simulink model "Single_Phase_FLL"  (R2021b)
settings: Solver=VariableStepAuto  StartTime=0.0  StopTime=2  RelTol=1e-3
libraries: dspswit3 x2, spsThreePhaseProgrammableVoltageSourceLib x1, spsThreePhaseVIMeasurementLib x1, spspowerguiLib x1
settings Model: Creator=Swaran Pratap Singh  LastModifiedBy=Swaran Pratap Singh
settings DataIOCC: InspectSignalLogs=on  ReturnWorkspaceOutputs=off

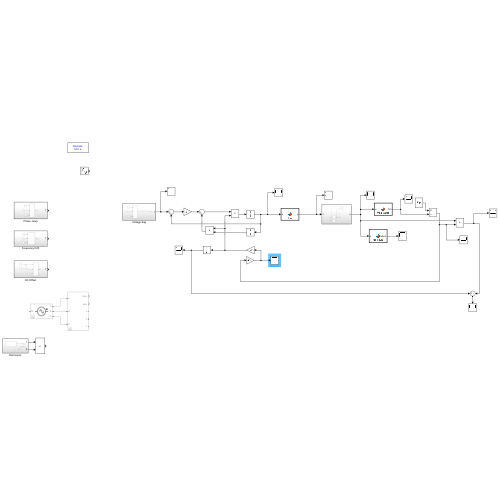
[thumbnail: Simulink's stored preview of the top-level diagram]
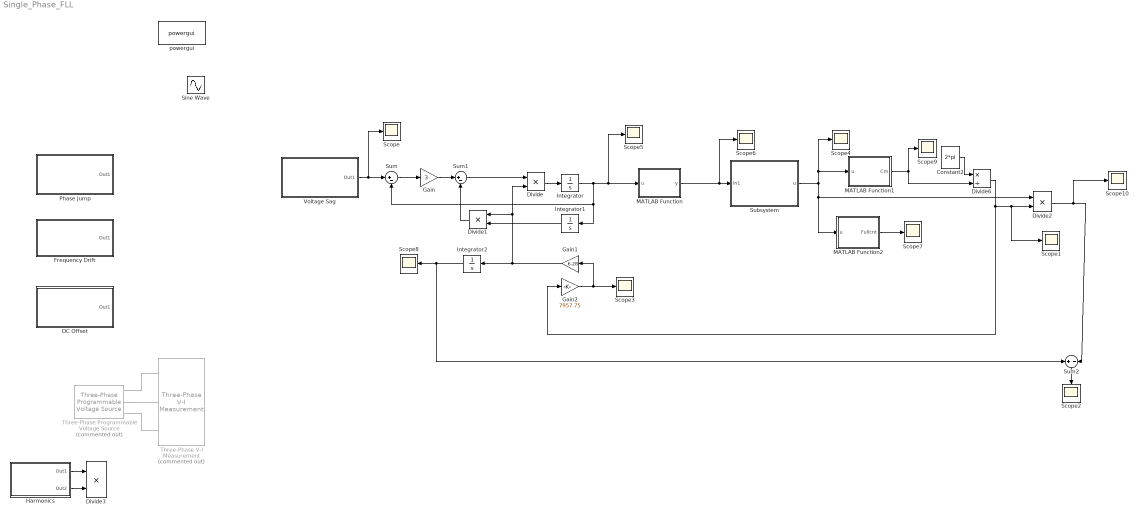
== system Single_Phase_FLL ==
  Constant2 : Constant  Value=2*pi
  DC Offset : Subsystem
  Divide{,1..3} (4 alike) : Product  Inputs=**
  Divide6 : Product  Inputs=*/
  Frequency Drift : Subsystem
  Gain : Gain  Gain=3
  Gain1 : Gain  Gain=6.28
  Gain2 : Gain  Gain=7957.75
  Harmonics : Subsystem
  Integrator : Integrator
  Integrator1 : Integrator
  Integrator2 : Integrator
  MATLAB Function : MATLAB Function  TreatAsAtomicUnit=on
  MATLAB Function1 : MATLAB Function  TreatAsAtomicUnit=on
  MATLAB Function2 : MATLAB Function  TreatAsAtomicUnit=on
  Phase Jump : Subsystem
  Scope{,1..10} (11 alike) : Scope
  Sine Wave : Sin  Amplitude=230  Frequency=2*pi*50  SampleTime=0.000001
  Subsystem : Subsystem
  Sum : Sum  Inputs=|+-
  Sum1 : Sum  Inputs=|+-
  Sum2 : Sum  Inputs=+-
  Three-Phase Programmable Voltage Source : spsThreePhaseProgrammableVoltageSourceLib/Three-Phase Programmable Voltage Source  Commented=on  PositiveSequence="[230  0 50]"  VariationEntity=Amplitude  VariationType=Table of time-amplitude pairs  VariationTypeAlt=Step  VariationStep=0.5  VariationRate=10  VariationMagnitude=0.3  VariationFrequency=2  VariationTiming=[1 2]  VariationPhaseA=off  Amplitudes=[ 0.05 0.1 0.06 ]  TimeValues=[0.145 0.145 0.145]  HarmonicGeneration=off  HarmonicA=[3 0.2 -25 0]  HarmonicB=[2 0.15 35 2]  Timing="[0.05  3]"  BusType=swing  Pref=0  Qref=0  Qmin=-inf  Qmax=inf
  Three-Phase V-I Measurement : spsThreePhaseVIMeasurementLib/Three-Phase V-I Measurement  Commented=on  VoltageMeasurement=phase-to-ground  SetLabelV=off  LabelV=Vabc  Vpu=off  VpuLL=off  CurrentMeasurement=yes  SetLabelI=off  LabelI=Iabc  Ipu=off  Pbase=100e6  Vbase=500e3  OutputType=Complex  PhasorSimulation=off  PSBequivalent=0
  Voltage Sag : Subsystem
  powergui : spspowerguiLib/powergui  Priority=1  SimulationMode=Discrete  SampleTime=1e-2  frequency=60  Iterations=50  frequencyindice=50  Pbase=100e6  ErrMax=1e-4  UnitsV=kV  UnitsW=MW  buscounter=0  FunctionMessages=off  echomessages=off  EnableUseOfTLC=off  CurrentSourceSwitches=off  DisableSnubberDevices=off  DisableRonSwitches=off  DisableVfSwitches=off  DisplayEquations=off  AutomaticDiscreteSolvers=off  SolverType=Tustin/Backward Euler (TBE)  Interpol=off  ExternalGateDelay=off  methode=off  Ts=100  x0status=blocks  SPID=on  SwTol=0  HookPort=off  NonlinearTolerance=1e-4  nMaxIteration=100  ContinueOnMaxIteration=off  RestoreLinks=warning  ResistiveCurrentMeasurement=off  Frange=[0:2:500]  Ylog=off  Xlog=on  ShowGrid=off  save=off  variable=ZData  structure=0  ZoomFFT=off  StartTime=0.0  cycles=1  DisplayStyle=1  fundamental=60  FreqAxis=off  MaxFrequency=1000  frequencyindicesteady=1  RmsSteady=1  display=off
  wires:
  Harmonics/2(Out2) -> Divide3/2
  Harmonics/1(Out1) -> Divide3/1
  MATLAB Function/1(y) -> Scope6/1, Subsystem/1(In1)
  Subsystem/1(u) -> MATLAB Function1/1(u), Scope4/1, MATLAB Function2/1(u), Divide2/1
  Gain1/1 -> Integrator2/1, Divide1/1, Divide/2
  Sum/1 -> Gain/1
  Divide2/1 -> Scope10/1, Sum2/2
  Integrator1/1 -> Divide1/2
  Divide1/1 -> Sum1/2
  Gain/1 -> Sum1/1
  Constant2/1 -> Divide6/1
  MATLAB Function2/1(Fullcnt) -> Scope7/1
  Divide/1 -> Integrator/1
  Integrator2/1 -> Sum2/1, Scope8/1
  MATLAB Function1/1(Cm) -> Divide6/2, Scope9/1
  Gain2/1 -> Scope3/1, Gain1/1
  Sum2/1 -> Scope2/1
  Divide6/1 -> Gain2/1, Scope1/1, Divide2/2
  Sum1/1 -> Divide/1
  Integrator/1 -> Integrator1/1, Sum/2, Scope5/1, MATLAB Function/1(u)
  Voltage Sag/1(Out1) -> Scope/1, Sum/1
  connections:
  Three-Phase Programmable Voltage Source/RConn2 -- Three-Phase V-I Measurement/LConn2
  Three-Phase Programmable Voltage Source/RConn1 -- Three-Phase V-I Measurement/LConn1
  Three-Phase Programmable Voltage Source/RConn3 -- Three-Phase V-I Measurement/LConn3

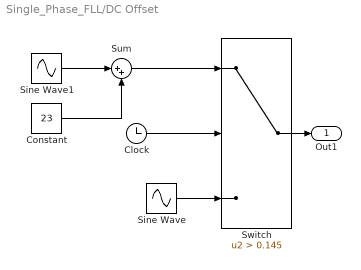
== system Single_Phase_FLL/DC Offset ==
  Clock : Clock
  Constant : Constant  Value=23
  Sine Wave : Sin  Amplitude=230  Frequency=314.16  SampleTime=0.000001
  Sine Wave1 : Sin  Amplitude=230  Frequency=314.16  SampleTime=0.000001
  Sum : Sum  Inputs=|++
  Switch : Switch  Criteria=u2 > Threshold  Threshold=0.145
  Out1 : Outport
  wires:
  Clock/1 -> Switch/2
  Sine Wave/1 -> Switch/3
  Switch/1 -> Out1/1
  Sine Wave1/1 -> Sum/1
  Constant/1 -> Sum/2
  Sum/1 -> Switch/1

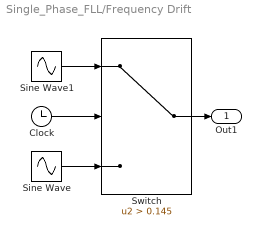
== system Single_Phase_FLL/Frequency Drift ==
  Clock : Clock
  Sine Wave : Sin  Amplitude=230  Frequency=314.16  SampleTime=0.000001
  Sine Wave1 : Sin  Amplitude=230  Frequency=333.01  Phase=pi  SampleTime=0.000001
  Switch : Switch  Criteria=u2 > Threshold  Threshold=0.145
  Out1 : Outport
  wires:
  Sine Wave1/1 -> Switch/1
  Sine Wave/1 -> Switch/3
  Clock/1 -> Switch/2
  Switch/1 -> Out1/1

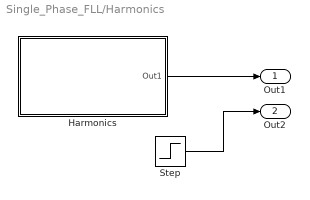
== system Single_Phase_FLL/Harmonics ==
  Harmonics : Subsystem
  Step : Step  Time=0  Before=230  After=230  SampleTime=0.000001
  Out1 : Outport
  Out2 : Outport  Port=2
  wires:
  Harmonics/1(Out1) -> Out1/1
  Step/1 -> Out2/1

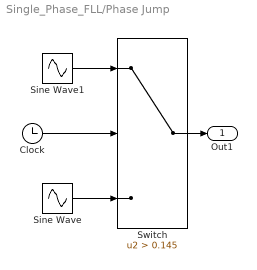
== system Single_Phase_FLL/Phase Jump ==
  Clock : Clock
  Sine Wave : Sin  Amplitude=230  Frequency=314.16  SampleTime=0.000001
  Sine Wave1 : Sin  Amplitude=230  Frequency=314.16  Phase=0.4167*pi  SampleTime=0.000001
  Switch : Switch  Criteria=u2 > Threshold  Threshold=0.145
  Out1 : Outport
  wires:
  Clock/1 -> Switch/2
  Sine Wave1/1 -> Switch/1
  Sine Wave/1 -> Switch/3
  Switch/1 -> Out1/1

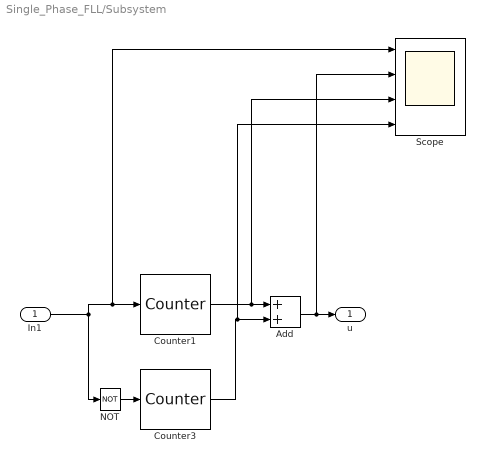
== system Single_Phase_FLL/Subsystem ==
  In1 : Inport
  Add : Sum
  Counter1 : dspswit3/Counter  Direction=Up  CountEvent=Free running  CounterSize=User defined  MaxCount=10000  InitialCount=0  Output=Count  HitValue=32  ResetInput=on  SamplesPerFrame=1  Ts=0.00001  CntDtype=double  HitDtype=Logical
  Counter3 : dspswit3/Counter  Direction=Up  CountEvent=Free running  CounterSize=User defined  MaxCount=10000  InitialCount=0  Output=Count  HitValue=32  ResetInput=on  SamplesPerFrame=1  Ts=0.00001  CntDtype=double  HitDtype=Logical
  NOT : Logic  Operator=NOT  IconShape=distinctive  AllPortsSameDT=off  OutDataTypeStr=boolean
  Scope : Scope  NumInputPorts=4
  u : Outport
  wires:
  NOT/1 -> Counter3/1
  Counter3/1 -> Scope/4, Add/2
  Counter1/1 -> Scope/3, Add/1
  In1/1 -> NOT/1, Scope/1, Counter1/1
  Add/1 -> Scope/2, u/1

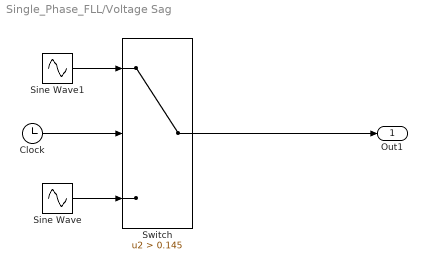
== system Single_Phase_FLL/Voltage Sag ==
  Clock : Clock
  Sine Wave : Sin  Amplitude=230  Frequency=314.16  SampleTime=0.000001
  Sine Wave1 : Sin  Amplitude=138  Frequency=314.16  SampleTime=0.000001
  Switch : Switch  Criteria=u2 > Threshold  Threshold=0.145
  Out1 : Outport
  wires:
  Clock/1 -> Switch/2
  Sine Wave1/1 -> Switch/1
  Sine Wave/1 -> Switch/3
  Switch/1 -> Out1/1

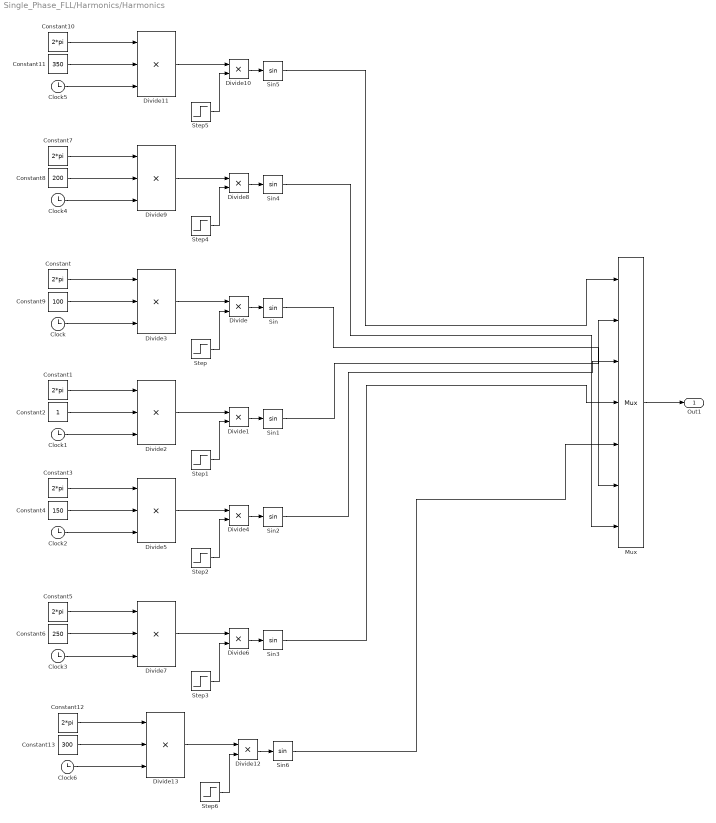
== system Single_Phase_FLL/Harmonics/Harmonics ==
  Clock{,1..6} (7 alike) : Clock
  Constant{,1,3,5,7,10,12} (7 alike) : Constant  Value=2*pi
  Constant11 : Constant  Value=350
  Constant13 : Constant  Value=300
  Constant2 : Constant
  Constant4 : Constant  Value=150
  Constant6 : Constant  Value=250
  Constant8 : Constant  Value=200
  Constant9 : Constant  Value=100
  Divide{,1,4,6,8,10,12} (7 alike) : Product  Inputs=**
  Divide{2..3,5,7,9,11,13} (7 alike) : Product  Inputs=***
  Mux : Mux  Inputs=7
  Sin{,1..6} (7 alike) : Trigonometry
  Step : Step  Time=0.145  Before=230  After=11.5  SampleTime=0.000001
  Step1 : Step  Time=0.145  Before=230  After=23  SampleTime=0.000001
  Step2 : Step  Time=0.145  Before=230  After=23  SampleTime=0.000001
  Step3 : Step  Time=0.145  Before=230  After=23  SampleTime=0.000001
  Step4 : Step  Time=0.145  Before=230  After=11.5  SampleTime=0.000001
  Step5 : Step  Time=0.145  Before=230  After=13.8  SampleTime=0.000001
  Step6 : Step  Time=0.145  Before=230  After=6.9  SampleTime=0.000001
  Out1 : Outport
  wires:
  Constant9/1 -> Divide3/2
  Clock/1 -> Divide3/3
  Constant/1 -> Divide3/1
  Divide3/1 -> Divide/1
  Divide/1 -> Sin/1
  Step/1 -> Divide/2
  Step1/1 -> Divide1/2
  Clock1/1 -> Divide2/3
  Constant1/1 -> Divide2/1
  Divide2/1 -> Divide1/1
  Constant2/1 -> Divide2/2
  Divide1/1 -> Sin1/1
  Constant3/1 -> Divide5/1
  Clock2/1 -> Divide5/3
  Divide4/1 -> Sin2/1
  Step2/1 -> Divide4/2
  Constant4/1 -> Divide5/2
  Divide5/1 -> Divide4/1
  Constant5/1 -> Divide7/1
  Clock3/1 -> Divide7/3
  Divide6/1 -> Sin3/1
  Step3/1 -> Divide6/2
  Constant6/1 -> Divide7/2
  Divide7/1 -> Divide6/1
  Step4/1 -> Divide8/2
  Constant8/1 -> Divide9/2
  Clock4/1 -> Divide9/3
  Divide8/1 -> Sin4/1
  Constant7/1 -> Divide9/1
  Divide9/1 -> Divide8/1
  Step5/1 -> Divide10/2
  Constant11/1 -> Divide11/2
  Clock5/1 -> Divide11/3
  Divide10/1 -> Sin5/1
  Constant10/1 -> Divide11/1
  Divide11/1 -> Divide10/1
  Step6/1 -> Divide12/2
  Constant13/1 -> Divide13/2
  Clock6/1 -> Divide13/3
  Divide12/1 -> Sin6/1
  Constant12/1 -> Divide13/1
  Divide13/1 -> Divide12/1
  Sin6/1 -> Mux/5
  Sin3/1 -> Mux/4
  Sin2/1 -> Mux/3
  Sin1/1 -> Mux/2
  Sin/1 -> Mux/6
  Sin4/1 -> Mux/7
  Sin5/1 -> Mux/1
  Mux/1 -> Out1/1

== matlab function Single_Phase_FLL/MATLAB Function1 ==
  data: u input; Cm output
function Cm = max_value(u)

persistent pre_u
persistent Cm_prev
flag = 1; % Remove int8 and initialization

if isempty(pre_u)
    pre_u = 1;
    Cm_prev=1;
end

if (pre_u > u)
    %Cm = pre_u;
    flag = 0;
else 
    %Cm = u;
    flag = 1;
end
%pre_u = Cm;
if (flag == 0)
    Cm = pre_u;
    Cm_prev=Cm;
    pre_u=u;
    flag = 1;
else
    pre_u=u;
    if(Cm_prev~=1)

        Cm=Cm_prev;
    else 
        Cm=pre_u;
    end
end
   
end

== matlab function Single_Phase_FLL/MATLAB Function ==
  data: u input; y output
function y = fcn(u)
    if u > 0
        y = 1;
    else
       y = 0;
    end
end

== matlab function Single_Phase_FLL/MATLAB Function2 ==
  data: u input; Fullcnt output
function   Fullcnt = full_count(u)

persistent pre_u
persistent Cm_prev
persistent cnt  
persistent Cm
flag = 1; % Remove int8 and initialization

if isempty(pre_u)
    pre_u = -1;
    Cm_prev=1;
    cnt=0;
    
end

if (pre_u > u)
    %Cm = pre_u;
    flag = 0;
else 
    %Cm = u;
    flag = 1;
end
%pre_u = Cm;
if (flag == 0)
    if(mod(cnt,2)==0)
        Cm = pre_u;
        Cm_prev=Cm;
    else
        Cm=Cm_prev;
    end
    pre_u=u;
    flag = 1;
    cnt=cnt+1;
else
    pre_u=u;
    if(Cm_prev~=1)

        Cm=Cm_prev;
    else 
    
            Cm=pre_u;

    end
end
if(mod(cnt,2)==1)
    Fullcnt=u+Cm;
else
    Fullcnt=u;
end
   
end
